simulink model "Simulation"  (R2024b)
settings: Solver=FixedStepAuto  StartTime=0.0  StopTime=inf  RelTol=1e-3
model workspace (MAT data in the model file):
  TimeOfDay = 560
  WeatherID = 6
settings Model: DataDictionary=DataDictionary.sldd  Creator=csamak  LastModifiedBy=tsamak
settings OptimizationCC: ZeroExternalMemoryAtStartup=off  ZeroInternalMemoryAtStartup=off  InitFltsAndDblsToZero=on
settings HardwareCC: ProdLongLongMode=on  TargetLongLongMode=on
settings SFSimCC: SimTargetLang=C++
settings RTWCC: TargetLang=C++  GenerateGPUCode=CUDA
settings GRTTargetCC: TargetLangStandard=C++11 (ISO)  CodeInterfacePackaging=C++ class

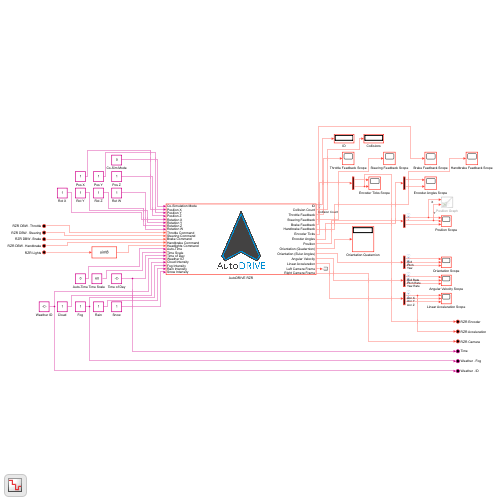
[thumbnail: Simulink's stored preview of the top-level diagram]
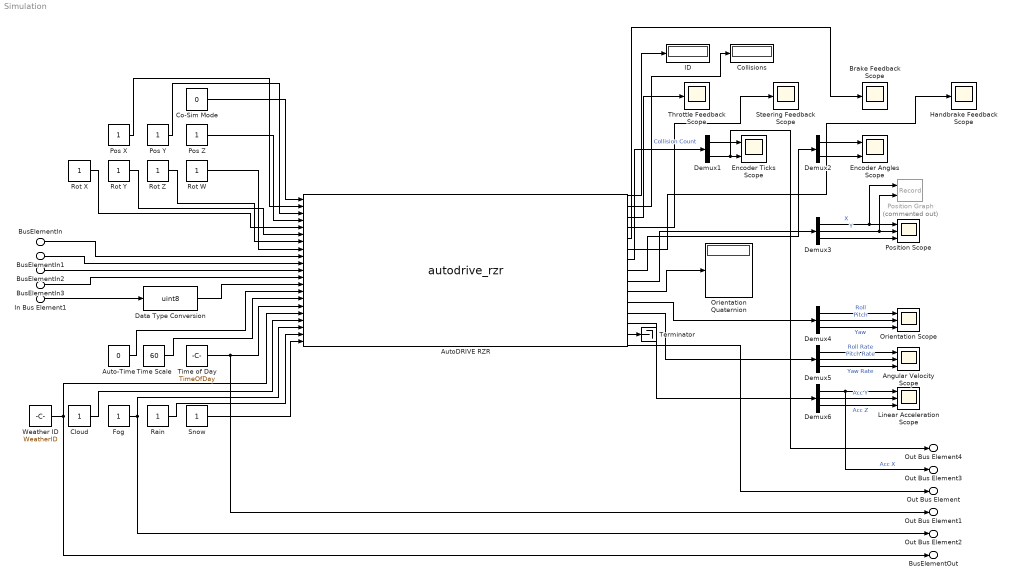
== system Simulation ==
  BusElementIn : Inport  PortName=RZR DBW  Element=Throttle
  BusElementIn1 : Inport  PortName=RZR DBW  Element=Steering
  BusElementIn2 : Inport  PortName=RZR DBW  Element=Brake
  BusElementIn3 : Inport  PortName=RZR DBW  Element=Handbrake
  In Bus Element1 : Inport  Port=2  PortName=RZR Lights
  Angular Velocity Scope : Scope  NumInputPorts=3
  Auto-Time : Constant  Value=0  OutDataTypeStr=boolean
  AutoDRIVE RZR : M-S-Function  FunctionName=autodrive_rzr  Parameters=Port  mask{Port=4567}
      mask Display:
      | image('autodrive_logo.png');
      | port_label('input', 1, 'Co-Simulation Mode');
      | port_label('input', 2, 'Position X');
      | port_label('input', 3, 'Position Y');
      | port_label('input', 4, 'Position Z');
      | port_label('input', 5, 'Rotation X');
      | port_label('input', 6, 'Rotation Y');
      | port_label('input', 7, 'Rotation Z');
      | port_label('input', 8, 'Rotation W');
      | port_label('input', 9, 'Throttle Command');
      | port_label('input', 10, 'Steering Command');
      | port_label('input', 11, 'Brake Command');
      | port_label('input', 12, 'Handbrake Command');
      | port_label('input', 13, 'Headlights Command');
      | port_label('input', 14, 'Auto-Time');
      | port_label('input', 15, 'Time Scale');
      | port_label('input', 16, 'Time of Day');
      | port_label('input', 17, 'Weather ID');
      | port_label('input', 18, 'Cloud Intensity');
      | port_label('input', 19, 'Fog Intensity');
      | port_label('input', 20, 'Rain Intensity');
      | port_label('input', 21, 'Snow Intensity');
      | port_label('output', 1, 'ID');
      | port_label('output', 2, 'Collision Count');
      | port_label('output', 3, 'Throttle Feedback');
      | port_label('output', 4, 'Steering Feedback');
      | port_label('output', 5, 'Brake Feedback');
      | port_label('output', 6, 'Handbrake Feedback');
      | port_label('output', 7, 'Encoder Ticks');
      | port_label('output', 8, 'Encoder Angles');
      | port_label('output', 9, 'Position');
      | port_label('output', 10, 'Orientation (Quaternion)');
      | port_label('output', 11, 'Orientation (Euler Angles)');
      | port_label('output', 12, 'Angular Velocity');
      | port_label('output', 13, 'Linear Acceleration');
      | port_label('output', 14, 'Left Camera Frame');
      | port_label('output', 15, 'Right Camera Frame');
  Brake Feedback Scope : Scope
  Cloud : Constant
  Co-Sim Mode : Constant  Value=0  OutDataTypeStr=uint8
  Collisions : Display
  Data Type Conversion : DataTypeConversion  OutDataTypeStr=uint8  RndMeth=Nearest  SaturateOnIntegerOverflow=off
  Demux1 : Demux  Outputs=2
  Demux2 : Demux  Outputs=2
  Demux{3..6} (4 alike) : Demux  Outputs=3
  Encoder Angles Scope : Scope  NumInputPorts=2
  Encoder Ticks Scope : Scope  NumInputPorts=2
  Fog : Constant
  Handbrake Feedback Scope : Scope
  ID : Display
  Linear Acceleration Scope : Scope  NumInputPorts=3
  Orientation Quaternion : Display
  Orientation Scope : Scope  NumInputPorts=3
  Pos X : Constant
  Pos Y : Constant
  Pos Z : Constant
  Position Graph : Record  Commented=on  FileSettingsInternal="{\"entries\":[{\"content\":{\"excelSettings\":{\"content\":{},\"type\":\"Streamout.ExcelSettings\"}},\"type\":\"Streamout.FileSettingStorage\",\"uuid\":\"\"}],\"packageUris\":[\"http:\\/\\/schema.mathworks.com\\/mf0\\/streamout_blocks\\/R2020a\"],\"version\":\"1.0\"}"  Layout=[1 1]  SignalsInternal="{\"entries\":[{\"content\":{},\"type\":\"RecordBlkView.InputSignals\",\"uuid\":\"\"}],\"packageUris\":[\"http:\\/\\/schema.mathworks.com\\/mf0\\/streamout_blocks\\/R2020a\"],\"version\":\"1.0\"}"  VisualizationBindings="{\"xyplotplugin\":{\"info\":[{\"series\":[],\"subplotID\":1}]}}"  CompatibilityTag=XY
  Position Scope : Scope  NumInputPorts=3
  Rain : Constant
  Rot W : Constant
  Rot X : Constant
  Rot Y : Constant
  Rot Z : Constant
  Snow : Constant
  Steering Feedback Scope : Scope
  Terminator : Terminator
  Throttle Feedback Scope : Scope
  Time Scale : Constant  Value=60
  Time of Day : Constant  Value=TimeOfDay  OutDataTypeStr=double
  Weather ID : Constant  Value=WeatherID  OutDataTypeStr=uint8
  Out Bus Element : Outport  PortName=RZR Camera
  Out Bus Element1 : Outport  Port=2  PortName=Time
  BusElementOut : Outport  Port=3  PortName=Weather  Element=ID
  Out Bus Element2 : Outport  Port=3  PortName=Weather  Element=Fog
  Out Bus Element3 : Outport  Port=4  PortName=RZR Acceleration
  Out Bus Element4 : Outport  Port=5  PortName=RZR Encoder
  wires:
  Time Scale/1 -> AutoDRIVE RZR/15
  Rot X/1 -> AutoDRIVE RZR/5
  BusElementIn1/1 -> AutoDRIVE RZR/10
  AutoDRIVE RZR/3 -> Throttle Feedback Scope/1
  Demux3/3 -> Position Scope/3
  AutoDRIVE RZR/4 -> Steering Feedback Scope/1
  Demux4/3 -> Orientation Scope/3  "Yaw"
  Rain/1 -> AutoDRIVE RZR/20
  Demux4/1 -> Orientation Scope/1  "Roll"
  AutoDRIVE RZR/12 -> Demux5/1
  BusElementIn/1 -> AutoDRIVE RZR/9
  Demux3/2 -> Position Scope/2, Position Graph/2  "Y"
  Demux5/2 -> Angular Velocity Scope/2  "Pitch Rate"
  BusElementIn3/1 -> AutoDRIVE RZR/12
  Snow/1 -> AutoDRIVE RZR/21
  AutoDRIVE RZR/11 -> Demux4/1
  BusElementIn2/1 -> AutoDRIVE RZR/11
  Cloud/1 -> AutoDRIVE RZR/18
  Pos Z/1 -> AutoDRIVE RZR/4
  Rot W/1 -> AutoDRIVE RZR/8
  Auto-Time/1 -> AutoDRIVE RZR/14
  Pos X/1 -> AutoDRIVE RZR/2
  Fog/1 -> Out Bus Element2/1, AutoDRIVE RZR/19
  AutoDRIVE RZR/8 -> Demux2/1
  Demux6/2 -> Linear Acceleration Scope/2  "Acc Y"
  Demux1/1 -> Encoder Ticks Scope/1
  AutoDRIVE RZR/2 -> Collisions/1  "Collision Count"
  AutoDRIVE RZR/6 -> Handbrake Feedback Scope/1
  Demux1/2 -> Out Bus Element4/1, Encoder Ticks Scope/2
  Demux5/3 -> Angular Velocity Scope/3  "Yaw Rate"
  Demux3/1 -> Position Scope/1, Position Graph/1  "X"
  AutoDRIVE RZR/10 -> Orientation Quaternion/1
  Demux5/1 -> Angular Velocity Scope/1  "Roll Rate"
  Rot Y/1 -> AutoDRIVE RZR/6
  Weather ID/1 -> BusElementOut/1, AutoDRIVE RZR/17
  Demux6/3 -> Linear Acceleration Scope/3  "Acc Z"
  Co-Sim Mode/1 -> AutoDRIVE RZR/1
  In Bus Element1/1 -> Data Type Conversion/1
  Demux2/2 -> Encoder Angles Scope/2
  AutoDRIVE RZR/13 -> Demux6/1
  Rot Z/1 -> AutoDRIVE RZR/7
  Demux6/1 -> Linear Acceleration Scope/1, Out Bus Element3/1  "Acc X"
  Demux4/2 -> Orientation Scope/2  "Pitch"
  Demux2/1 -> Encoder Angles Scope/1
  Pos Y/1 -> AutoDRIVE RZR/3
  AutoDRIVE RZR/5 -> Brake Feedback Scope/1
  AutoDRIVE RZR/7 -> Demux1/1
  AutoDRIVE RZR/1 -> ID/1
  AutoDRIVE RZR/9 -> Demux3/1
  AutoDRIVE RZR/15 -> Out Bus Element/1
  Time of Day/1 -> Out Bus Element1/1, AutoDRIVE RZR/16
  AutoDRIVE RZR/14 -> Terminator/1
  Data Type Conversion/1 -> AutoDRIVE RZR/13
